simulink model "Reference_Signals"  (R2019b)
settings: Solver=VariableStepAuto  StartTime=0.0  StopTime=500  RelTol=1e-3
settings Model: Creator=OPAL_PC  LastModifiedBy=OPAL_PC

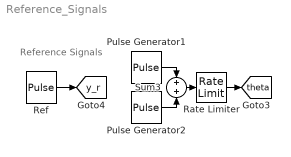
== system Reference_Signals ==
  note: Reference Signals
  Pulse Generator1 : DiscretePulseGenerator  PulseType=Time based  Period=200  PulseWidth=50
  Pulse Generator2 : DiscretePulseGenerator  PulseType=Time based  Amplitude=-1  Period=200  PulseWidth=50  PhaseDelay=50
  Rate Limiter : RateLimiter  RisingSlewLimit=0.05  FallingSlewLimit=-0.05  SampleTimeMode=inherited
  Ref : DiscretePulseGenerator  PulseType=Time based  Amplitude=0.5  Period=10  PulseWidth=50
  Sum3 : Sum
  tag scope: theta=global, y_r=global
  wires:
  Pulse Generator1/1 -> Sum3/1
  Sum3/1 -> Rate Limiter/1
  Pulse Generator2/1 -> Sum3/2
  Rate Limiter/1 -> [theta]
  Ref/1 -> [y_r]
